simulink model "PH3_CSI_spv"  (R2017a)
settings: Solver=VariableStepAuto  StartTime=0.0  StopTime=10.0  MaxStep=1e-4  RelTol=1e-3
undefined symbols (not defined in the file): st_time3
libraries: powerlib x32, powerlib_meascontrol x6
settings Model: Creator=erich  LastModifiedBy=erich

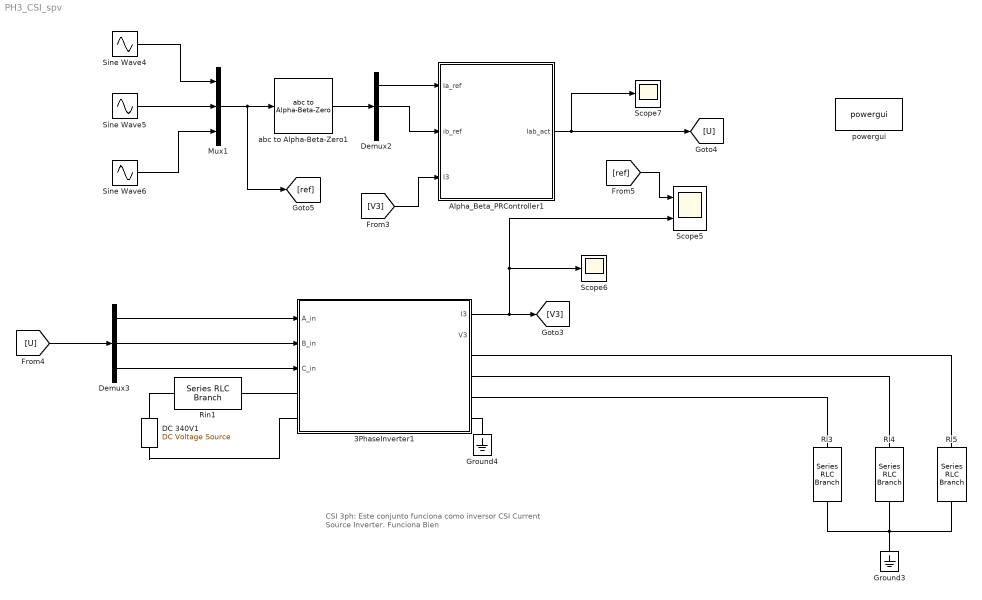
== system PH3_CSI_spv ==
  note: CSI 3ph:
      | Este conjunto funciona como inversor CSI
      | Current Source Inverter. Funciona Bien
  3PhaseInverter1 : Subsystem  mask{f_sw=10000, start_Delay=2e-3}
      mask prompts: f_sw "Switching Frequency (Hz)"; start_Delay "Time delay for drivers (s)"
      mask Display:
      | port_label('input', 1, 'A_u', 'texmode', 'on')
      | port_label('input', 2, 'B_u', 'texmode', 'on')
      | port_label('input', 3, 'C_u', 'texmode', 'on')
      | 
      | port_label('lconn', 1, 'DC +')
      | port_label('lconn', 2, 'DC -')
      | 
      | 
      | port_label('rconn', 1, 'A')
      | port_label('rconn', 2, 'B')
      | port_label('rconn', 3, 'C')
      | port_label('rconn', 4, 'Neutral')
      | 
      | port_label('output', 1, 'I_{3\Phi}', 'texmode', 'on')
      | port_label('output', 2, 'V_{3\Phi}', 'texmode', 'on')
      | 
      | plot([0.1 .9], [0.1 .9])
      | plot([0.2 .4], [.7 .7])
      | plot([0.2 .24], [.65 .65])
      | plot([0.28 .32], [.65 .65])
      | plot([0.36 .40], [.65 .65])
      | 
      | plot([.5:.01:.7], .25+sin(30*[.2:.01:.4])/10)
  Alpha_Beta_PRController1 : Subsystem  mask{Kp=50/100, Ki=25, w0=2*pi*60, wa=10}
      mask prompts: Kp "Ganancia Proporcional"; Ki "Ganancia Integral"; w0 "Frencuencia Central"; wa "Ancho de campana de resonancia"
      mask Display:
      | port_label('input', 1, '\fontsize{13} \alpha_{ref}', 'texmode', 'on')
      | port_label('input', 2, '\fontsize{13} \beta_{ref}', 'texmode', 'on')
      | port_label('input', 3, '\fontsize{13} [ a, b, c ]', 'texmode', 'on')
      | 
      | port_label('output', 1, '\fontsize{13} [ u_{a}, u_{b}, u_{c} ]', 'texmode', 'on')
      | 
      | 
      | %plot([.4 .6],.05+[.5 .7])
      | %plot([.4 .6],.05+[.9 .7])
      | %plot([.4 .4],.05+[.9 .5])
      | 
      | text(.53,.2,'\fontsize{25} \int', 'texmode', 'on')
      | plot(.65+[0:.01:pi/10], .2+sin(40*[0:.01:pi/10])/13)
      | 
      | %text(.5,.8,'\fontsize{15} PR_{\alpha \beta}', 'texmode', 'on')
  DC 340V1 : powerlib/Electrical Sources/DC Voltage Source  Amplitude=1000  Measurements=None
  Demux2 : Demux  Outputs=3
  Demux3 : Demux  Outputs=3
  Ground3 : powerlib/Elements/Ground  LConnTagsString=a
  Ground4 : powerlib/Elements/Ground  LConnTagsString=a
  Mux1 : Mux  Inputs=3
  Rin1 : powerlib/Elements/Series RLC Branch  LConnTagsString=__new0  RConnTagsString=__new0  BranchType=R  Resistance=.01  Inductance=0  SetiL0=off  InitialCurrent=0  Capacitance=0  Setx0=off  InitialVoltage=0  Measurements=None
  Rl3 : powerlib/Elements/Series RLC Branch  LConnTagsString=__new0  RConnTagsString=__new0  BranchType=R  Resistance=50  Inductance=1e-3  SetiL0=off  InitialCurrent=0  Capacitance=1e-6  Setx0=off  InitialVoltage=0  Measurements=None
  Rl4 : powerlib/Elements/Series RLC Branch  LConnTagsString=__new0  RConnTagsString=__new0  BranchType=R  Resistance=50  Inductance=1e-3  SetiL0=off  InitialCurrent=0  Capacitance=1e-6  Setx0=off  InitialVoltage=0  Measurements=None
  Rl5 : powerlib/Elements/Series RLC Branch  LConnTagsString=__new0  RConnTagsString=__new0  BranchType=R  Resistance=50  Inductance=1e-3  SetiL0=off  InitialCurrent=0  Capacitance=1e-6  Setx0=off  InitialVoltage=0  Measurements=None
  Scope5 : Scope  NumInputPorts=2
  Scope6 : Scope
  Scope7 : Scope
  Sine Wave4 : Sin  Amplitude=10  Frequency=2*pi*60
  Sine Wave5 : Sin  Amplitude=10  Frequency=2*pi*60  Phase=2*pi/3
  Sine Wave6 : Sin  Amplitude=10  Frequency=2*pi*60  Phase=-2*pi/3
  abc to Alpha-Beta-Zero1 : powerlib_meascontrol/Transformations/abc to Alpha-Beta-Zero
      settings: SourceProductName=Simscape Power Systems
  powergui : powerlib/powergui  Priority=1  SimulationMode=Continuous  SampleTime=50e-6  frequency=60  Iterations=50  frequencyindice=0  Pbase=100e6  ErrMax=1e-4  UnitsV=kV  UnitsW=MW  buscounter=0  FunctionMessages=off  echomessages=off  EnableUseOfTLC=off  CurrentSourceSwitches=off  DisableSnubberDevices=off  DisableRonSwitches=off  DisableVfSwitches=off  DisplayEquations=off  SolverType=Tustin/Backward Euler (TBE)  Interpol=off  ExternalGateDelay=off  methode=off  Ts=100  x0status=blocks  SPID=on  SwTol=0  HookPort=off  RestoreLinks=warning  ResistiveCurrentMeasurement=off  Frange=[0:2:500]  Ylog=off  Xlog=on  ShowGrid=off  save=off  variable=ZData  structure=0  ZoomFFT=off  StartTime=0.0  cycles=1  DisplayStyle=1  fundamental=60  FreqAxis=off  MaxFrequency=1000  frequencyindicesteady=1  RmsSteady=1  display=off
  wires:
  Demux3/3 -> 3PhaseInverter1/3(C_in)
  Demux2/2 -> Alpha_Beta_PRController1/2(ib_ref)
  Sine Wave4/1 -> Mux1/1
  3PhaseInverter1/1(I3) -> [V3], Scope6/1, Scope5/2
  Sine Wave6/1 -> Mux1/3
  [V3] -> Alpha_Beta_PRController1/3(I3)
  Mux1/1 -> abc to Alpha-Beta-Zero1/1, [ref]
  [ref] -> Scope5/1
  Demux2/1 -> Alpha_Beta_PRController1/1(Ia_ref)
  abc to Alpha-Beta-Zero1/1 -> Demux2/1
  Sine Wave5/1 -> Mux1/2
  Demux3/2 -> 3PhaseInverter1/2(B_in)
  Alpha_Beta_PRController1/1(Iab_act) -> [U], Scope7/1
  Demux3/1 -> 3PhaseInverter1/1(A_in)
  [U] -> Demux3/1
  connections:
  Rl4/RConn1 -- Rl5/RConn1 -- Ground3/LConn1 -- Rl3/RConn1
  Rl3/LConn1 -- 3PhaseInverter1/RConn3
  Rin1/RConn1 -- 3PhaseInverter1/LConn1
  Rl5/LConn1 -- 3PhaseInverter1/RConn1
  DC 340V1/RConn1 -- Rin1/LConn1
  Rl4/LConn1 -- 3PhaseInverter1/RConn2
  DC 340V1/LConn1 -- 3PhaseInverter1/LConn2
  3PhaseInverter1/RConn4 -- Ground4/LConn1

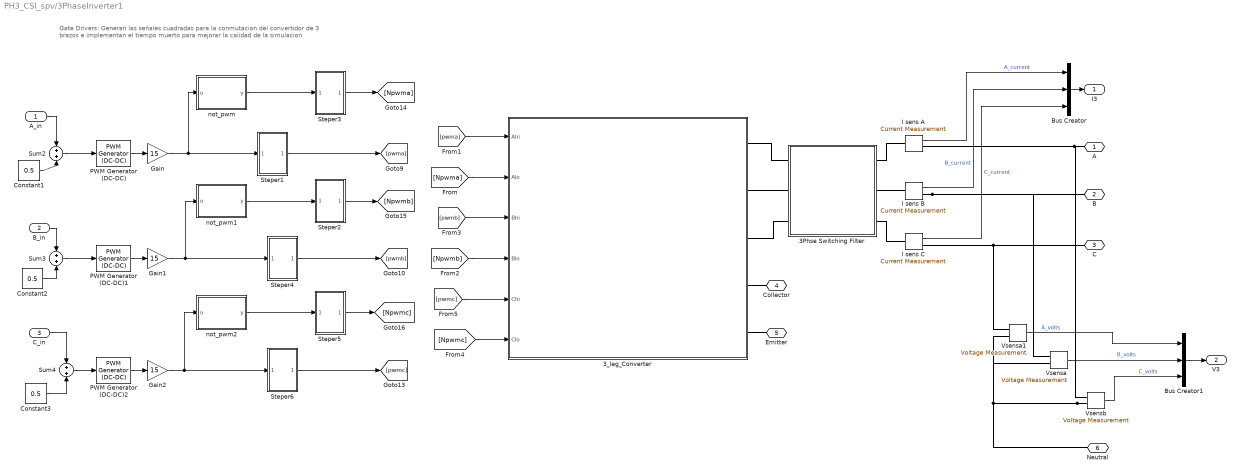
== system PH3_CSI_spv/3PhaseInverter1 ==
  note: Gate Drivers: Generan las señales cuadradas para
      | la conmutacion del convertidor de 3 brazos e implementan el
      | tiempo muerto para mejorar la calidad de la simulacion
  A_in : Inport
  B_in : Inport  Port=2
  C_in : Inport  Port=3
  3Phse Switching Filter : Subsystem
      mask Display:
      | port_label('lconn', 1, 'A_{in}', 'texmode', 'on')
      | port_label('lconn', 2, 'B_{in}', 'texmode', 'on')
      | port_label('lconn', 3, 'B_{in}', 'texmode', 'on')
      | port_label('rconn', 1, 'A_{out}', 'texmode', 'on')
      | port_label('rconn', 2, 'B_{out}', 'texmode', 'on')
      | port_label('rconn', 3, 'C_{out}', 'texmode', 'on')
      | 
      | 
      | plot([.2 .5], [.7 .7])
      | plot([.5 .6], [.7 .3])
      | plot([.6 .7], [.3 .3])
      | 
      | text(.2, .8, '\fontsize{12} H(\omega)', 'texmode', 'on')
      | text(.6, .25, '\fontsize{12} \omega', 'texmode', 'on')
  3_leg_Converter : Subsystem
      mask Display:
      | port_label('input', 1, 'Ahi')
      | port_label('input', 2, 'Alo')
      | port_label('input', 3, 'Bhi')
      | port_label('input', 4, 'Blo')
      | port_label('input', 5, 'Chi')
      | port_label('input', 6, 'Clo')
      | 
      | port_label('rconn', 1, 'A')
      | port_label('rconn', 2, 'B')
      | port_label('rconn', 3, 'C')
      | port_label('rconn', 4, 'Collector')
      | port_label('rconn', 5, 'Emitter')
      | 
      | lvx = [.1 .1];
      | lvy = [.1 .2];
      | lhx = [.1 .2];
      | lhy = [.1 .1];
      | 
      | 
      | % se dibujan los interruptores de la izquierda
      | plot(lvx+.07, lvy*.8+.028+.1)
      | plot(lvx+.1, lvy+.1)
      | plot(lhx*.5+.15, lhy+.1)
      | plot(lhx*.5+.15, lhy+.2)
      | plot(lhx*.5+.07, lhy+.15)
      | 
      | d=0.5;
      | 
      | plot(lvx+.07, lvy*.8+.028+.1+d)
      | plot(lvx+.1, lvy+.1+d)
      | plot(lhx*.5+.15, lhy+.1+d)
      | plot(lhx*.5+.15, lhy+.2+d)
      | plot(lhx*.5+.07, lhy+.15+d)
      | 
      | 
      | % se dibujan los interruptores del medio
      | h=.3;
      | 
      | plot(lvx+.07+h, lvy*.8+.028+.1)
      | plot(lvx+.1+h, lvy+.1)
      | plot(lhx*.5+.15+h, lhy+.1)
      | plot(lhx*.5+.15+h, lhy+.2)
      | plot(lhx*.5+.07+h, lhy+.15)
      | 
      | plot(lvx+.07+h, lvy*.8+.028+.1+d)
      | plot(lvx+.1+h, lvy+.1+d)
      | plot(lhx*.5+.15+h, lhy+.1+d)
      | plot(lhx*.5+.15+h, lhy+.2+d)
      | plot(lhx*.5+.07+h, lhy+.15+d)
      | 
      | % se dibujan los interruptores de la derecha
      | h=.6
      | 
      | plot(lvx+.07+h, lvy*.8+.028+.1)
      | plot(lvx+.1+h, lvy+.1)
      | plot(lhx*.5+.15+h, lhy+.1)
      | plot(lhx*.5+.15+h, lhy+.2)
      | plot(lhx*.5+.07+h, lhy+.15)
      | 
      | plot(lvx+.07+h, lvy*.8+.028+.1+d)
      | plot(lvx+.1+h, lvy+.1+d)
      | plot(lhx*.5+.15+h, lhy+.1+d)
      | plot(lhx*.5+.15+h, lhy+.2+d)
      | plot(lhx*.5+.07+h, lhy+.15+d)
      | 
      | 
      | % se conectan los interruptores.
      | plot(lvx+.15, lvy*4-.1)
      | plot(lvx+.15+.3, lvy*4-.1)
      | plot(lvx+.15+.6, lvy*4-.1)
      | 
      | 
      | plot(lvx+.15, lvy+.7)
      | plot(lvx+.15+.3, lvy+.7)
      | plot(lvx+.15+.6, lvy+.7)
      | 
      | plot(lvx+.15, lvy)
      | plot(lvx+.15+.3, lvy)
      | plot(lvx+.15+.6, lvy)
      | 
      | plot(lhx*6-.35, lhy)
      | plot(lhx*6-.35, lhy+.8)
      | 
      | % raul esteban alzate 313 515 86 11
  Bus Creator : BusCreator  Inputs='A_current','B_current','C_current'
  Bus Creator1 : BusCreator  Inputs='A_volts','B_volts','C_volts'
  Constant1 : Constant  Value=0.5
  Constant2 : Constant  Value=0.5
  Constant3 : Constant  Value=0.5
  Gain : Gain  Gain=15
  Gain1 : Gain  Gain=15
  Gain2 : Gain  Gain=15
  I sens A : powerlib/Measurements/Current Measurement  PhasorSimulation=off  OutputType=Complex  PSBequivalent=0
  I sens B : powerlib/Measurements/Current Measurement  PhasorSimulation=off  OutputType=Complex  PSBequivalent=0
  I sens C : powerlib/Measurements/Current Measurement  PhasorSimulation=off  OutputType=Complex  PSBequivalent=0
  PWM Generator (DC-DC) : powerlib_meascontrol/Pulse & Signal Generators/PWM Generator (DC-DC)  Fsw=f_sw  Ts=0
  PWM Generator (DC-DC)1 : powerlib_meascontrol/Pulse & Signal Generators/PWM Generator (DC-DC)  Fsw=f_sw  Ts=0
  PWM Generator (DC-DC)2 : powerlib_meascontrol/Pulse & Signal Generators/PWM Generator (DC-DC)  Fsw=f_sw  Ts=0
  Steper1 : Subsystem
  Steper2 : Subsystem
  Steper3 : Subsystem
  Steper4 : Subsystem
  Steper5 : Subsystem
  Steper6 : Subsystem
  Sum2 : Sum
  Sum3 : Sum
  Sum4 : Sum
  Vsensa : powerlib/Measurements/Voltage Measurement  PhasorSimulation=off  OutputType=Complex  PSBequivalent=0
  Vsensa1 : powerlib/Measurements/Voltage Measurement  PhasorSimulation=off  OutputType=Complex  PSBequivalent=0
  Vsensb : powerlib/Measurements/Voltage Measurement  PhasorSimulation=off  OutputType=Complex  PSBequivalent=0
  not_pwm : MATLAB Function  TreatAsAtomicUnit=on
  not_pwm1 : MATLAB Function  TreatAsAtomicUnit=on
  not_pwm2 : MATLAB Function  TreatAsAtomicUnit=on
  A : PMIOPort  Port=1  Side=Right
  B : PMIOPort  Port=2  Side=Right
  C : PMIOPort  Port=3  Side=Right
  Collector : PMIOPort  Port=4  Side=Left
  Emitter : PMIOPort  Port=5  Side=Left
  Neutral : PMIOPort  Port=6  Side=Right
  I3 : Outport
  V3 : Outport  Port=2
  wires:
  [Npwmc] -> 3_leg_Converter/6(Clo)
  [pwmc] -> 3_leg_Converter/5(Chi)
  [Npwmb] -> 3_leg_Converter/4(Blo)
  [pwmb] -> 3_leg_Converter/3(Bhi)
  [Npwma] -> 3_leg_Converter/2(Alo)
  [pwma] -> 3_leg_Converter/1(Ahi)
  Vsensa1/1 -> Bus Creator1/1  "A_volts"
  Vsensa/1 -> Bus Creator1/2  "B_volts"
  Bus Creator1/1 -> V3/1
  Vsensb/1 -> Bus Creator1/3  "C_volts"
  Steper6/1(Out1) -> [pwmc]
  Gain/1 -> not_pwm/1(u), Steper1/1(In1)
  Steper3/1(Out1) -> [Npwma]
  Constant2/1 -> Sum3/2
  I sens B/1 -> Bus Creator/2  "B_current"
  Steper1/1(Out1) -> [pwma]
  Steper5/1(Out1) -> [Npwmc]
  Gain2/1 -> not_pwm2/1(u), Steper6/1(In1)
  Sum3/1 -> PWM Generator (DC-DC)1/1
  Bus Creator/1 -> I3/1
  I sens A/1 -> Bus Creator/1  "A_current"
  A_in/1 -> Sum2/1
  Steper2/1(Out1) -> [Npwmb]
  Constant1/1 -> Sum2/2
  B_in/1 -> Sum3/1
  PWM Generator (DC-DC)/1 -> Gain/1
  I sens C/1 -> Bus Creator/3  "C_current"
  Sum2/1 -> PWM Generator (DC-DC)/1
  C_in/1 -> Sum4/1
  not_pwm2/1(y) -> Steper5/1(In1)
  PWM Generator (DC-DC)1/1 -> Gain1/1
  Constant3/1 -> Sum4/2
  not_pwm/1(y) -> Steper3/1(In1)
  Sum4/1 -> PWM Generator (DC-DC)2/1
  PWM Generator (DC-DC)2/1 -> Gain2/1
  not_pwm1/1(y) -> Steper2/1(In1)
  Gain1/1 -> not_pwm1/1(u), Steper4/1(In1)
  Steper4/1(Out1) -> [pwmb]
  connections:
  3_leg_Converter/RConn5 -- Emitter/RConn1
  3_leg_Converter/RConn4 -- Collector/RConn1
  Vsensb/LConn2 -- Vsensa1/LConn2 -- Vsensa/LConn2 -- Neutral/RConn1
  I sens C/LConn1 -- 3Phse Switching Filter/RConn3
  C/RConn1 -- I sens C/RConn1 -- Vsensa1/LConn1
  3Phse Switching Filter/LConn1 -- 3_leg_Converter/RConn1
  I sens B/RConn1 -- Vsensa/LConn1 -- B/RConn1
  I sens A/LConn1 -- 3Phse Switching Filter/RConn1
  3Phse Switching Filter/LConn3 -- 3_leg_Converter/RConn3
  A/RConn1 -- I sens A/RConn1 -- Vsensb/LConn1
  I sens B/LConn1 -- 3Phse Switching Filter/RConn2
  3Phse Switching Filter/LConn2 -- 3_leg_Converter/RConn2

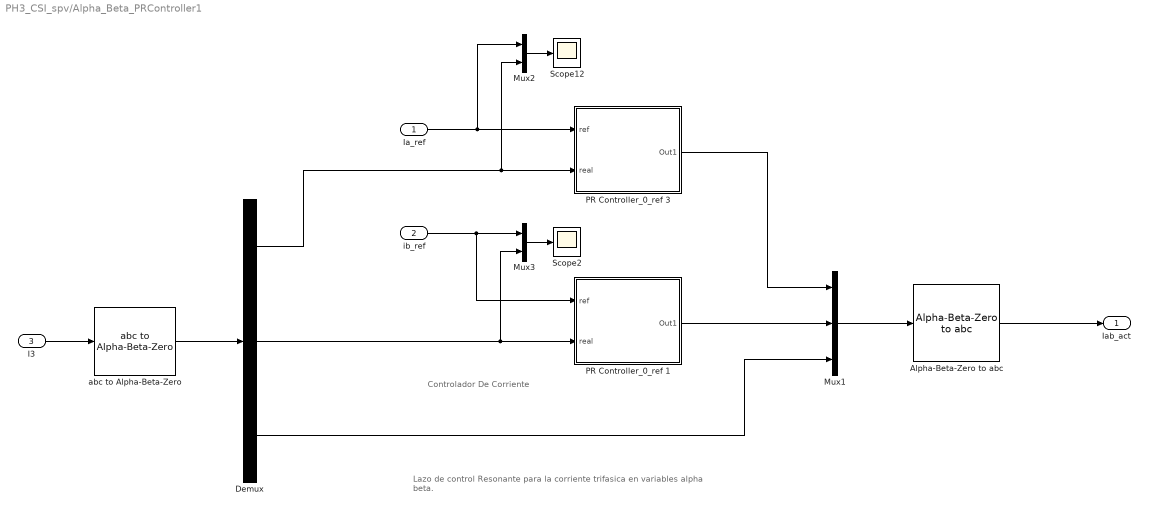
== system PH3_CSI_spv/Alpha_Beta_PRController1 ==
  note: Lazo de control Resonante para la
      | corriente trifasica en variables alpha beta.
  note: Controlador De Corriente
  Ia_ref : Inport
  ib_ref : Inport  Port=2
  I3 : Inport  Port=3
  Alpha-Beta-Zero to abc : powerlib_meascontrol/Transformations/Alpha-Beta-Zero to abc
      settings: SourceProductName=Simscape Power Systems  SourceProductBaseCode=PS
  Demux : Demux  Outputs=3
  Mux1 : Mux  Inputs=3
  Mux2 : Mux  Inputs=2
  Mux3 : Mux  Inputs=2
  PR Controller_0_ref 1 : Subsystem  mask{Kp=Kp, Ki=Ki, wa=wa, w0=w0}
      mask prompts: Kp "Ganancia Proporcional"; Ki "Ganancia Integral"; wa "Ancho camapana resonancia"; w0 "Frecuencia Central"
      mask Display:
      | port_label('input',1,'ref')
      | port_label('input',2,'sens')
      | port_label('output',1,'out')
      | 
      | plot(.4+[0:.01:pi/10], .32+sin(40*[0:.01:pi/10])/13)
      | 
      | plot([.4 .6],.05+[.5 .7])
      | plot([.4 .6],.05+[.9 .7])
      | plot([.4 .4],.05+[.9 .5])
      | 
      | text(.27,.37,'\fontsize{25} \int', 'texmode', 'on')
  PR Controller_0_ref 3 : Subsystem  mask{Kp=Kp, Ki=Ki, wa=wa, w0=w0}
      mask prompts: Kp "Ganancia Proporcional"; Ki "Ganancia Integral"; wa "Ancho camapana resonancia"; w0 "Frecuencia Central"
      mask Display:
      | port_label('input',1,'ref')
      | port_label('input',2,'sens')
      | port_label('output',1,'out')
      | 
      | plot(.4+[0:.01:pi/10], .32+sin(40*[0:.01:pi/10])/13)
      | 
      | plot([.4 .6],.05+[.5 .7])
      | plot([.4 .6],.05+[.9 .7])
      | plot([.4 .4],.05+[.9 .5])
      | 
      | text(.27,.37,'\fontsize{25} \int', 'texmode', 'on')
  Scope12 : Scope
  Scope2 : Scope
  abc to Alpha-Beta-Zero : powerlib_meascontrol/Transformations/abc to Alpha-Beta-Zero
      settings: SourceProductName=Simscape Power Systems
  Iab_act : Outport
  wires:
  Demux/1 -> PR Controller_0_ref 3/2(real), Mux2/2
  Demux/3 -> Mux1/3
  PR Controller_0_ref 3/1(Out1) -> Mux1/1
  Ia_ref/1 -> PR Controller_0_ref 3/1(ref), Mux2/1
  ib_ref/1 -> Mux3/1, PR Controller_0_ref 1/1(ref)
  abc to Alpha-Beta-Zero/1 -> Demux/1
  Alpha-Beta-Zero to abc/1 -> Iab_act/1
  Mux3/1 -> Scope2/1
  Mux1/1 -> Alpha-Beta-Zero to abc/1
  PR Controller_0_ref 1/1(Out1) -> Mux1/2
  Demux/2 -> Mux3/2, PR Controller_0_ref 1/2(real)
  Mux2/1 -> Scope12/1
  I3/1 -> abc to Alpha-Beta-Zero/1

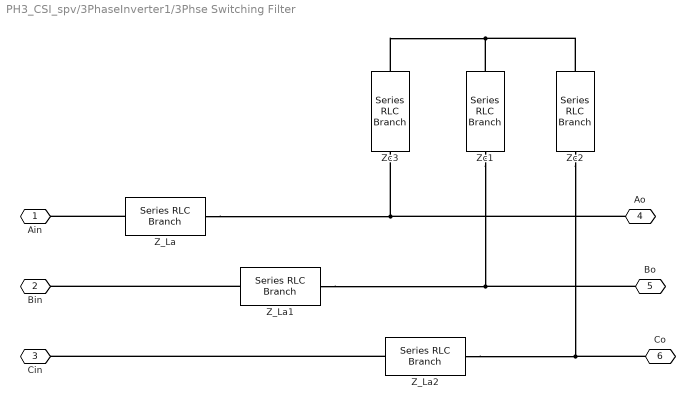
== system PH3_CSI_spv/3PhaseInverter1/3Phse Switching Filter ==
  Z_La : powerlib/Elements/Series RLC Branch  LConnTagsString=__new0  RConnTagsString=__new0  BranchType=RL  Resistance=.01  Inductance=4e-3  SetiL0=off  InitialCurrent=0  Capacitance=2.2e-6  Setx0=off  InitialVoltage=0  Measurements=None
  Z_La1 : powerlib/Elements/Series RLC Branch  LConnTagsString=__new0  RConnTagsString=__new0  BranchType=RL  Resistance=.1  Inductance=4e-3  SetiL0=off  InitialCurrent=0  Capacitance=2.2e-6  Setx0=off  InitialVoltage=0  Measurements=None
  Z_La2 : powerlib/Elements/Series RLC Branch  LConnTagsString=__new0  RConnTagsString=__new0  BranchType=RL  Resistance=.1  Inductance=4e-3  SetiL0=off  InitialCurrent=0  Capacitance=2.2e-6  Setx0=off  InitialVoltage=0  Measurements=None
  Zc1 : powerlib/Elements/Series RLC Branch  LConnTagsString=__new0  RConnTagsString=__new0  BranchType=RC  Resistance=1e-3  Inductance=1e-9  SetiL0=off  InitialCurrent=0  Capacitance=2.2e-6  Setx0=off  InitialVoltage=0  Measurements=None
  Zc2 : powerlib/Elements/Series RLC Branch  LConnTagsString=__new0  RConnTagsString=__new0  BranchType=RC  Resistance=1e-3  Inductance=1e-9  SetiL0=off  InitialCurrent=0  Capacitance=2.2e-6  Setx0=off  InitialVoltage=0  Measurements=None
  Zc3 : powerlib/Elements/Series RLC Branch  LConnTagsString=__new0  RConnTagsString=__new0  BranchType=RC  Resistance=1e-3  Inductance=1e-9  SetiL0=off  InitialCurrent=0  Capacitance=2.2e-6  Setx0=off  InitialVoltage=0  Measurements=None
  Ain : PMIOPort  Port=1  Side=Left
  Bin : PMIOPort  Port=2  Side=Left
  Cin : PMIOPort  Port=3  Side=Left
  Ao : PMIOPort  Port=4  Side=Right
  Bo : PMIOPort  Port=5  Side=Right
  Co : PMIOPort  Port=6  Side=Right
  connections:
  Z_La2/LConn1 -- Cin/RConn1
  Z_La1/LConn1 -- Bin/RConn1
  Z_La/LConn1 -- Ain/RConn1
  Z_La/RConn1 -- Zc3/LConn1 -- Ao/RConn1
  Z_La2/RConn1 -- Co/RConn1 -- Zc2/LConn1
  Z_La1/RConn1 -- Zc1/LConn1 -- Bo/RConn1
  Zc2/RConn1 -- Zc1/RConn1 -- Zc3/RConn1

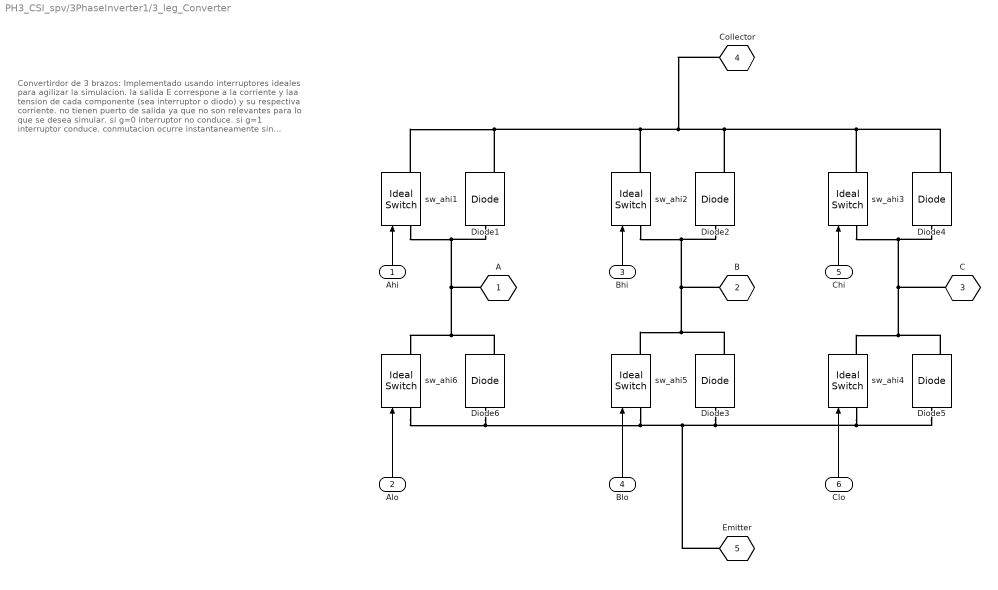
== system PH3_CSI_spv/3PhaseInverter1/3_leg_Converter ==
  note: Convertirdor de 3 brazos:
      |
      | Implementado usando interruptores
      | ideales para agilizar la simulacion.
      | la salida E correspone a la corriente y laa
      | tension de cada componente
      | (sea interruptor o diodo) y su respectiva
      | corriente. no tienen puerto de salida ya que no
      | son relevantes para lo que se desea simular.
      |
      | si g=0 interruptor no conduce.
      | si g=1 interruptor conduce.
      |
      | conmutacion ocurre instantaneamente sin
      | retardo.
  Ahi : Inport
  Alo : Inport  Port=2
  Bhi : Inport  Port=3
  Blo : Inport  Port=4
  Chi : Inport  Port=5
  Clo : Inport  Port=6
   sw_ahi{1..6} (6 alike) : powerlib/Power Electronics/Ideal Switch  Ron=20e-3  Lon=0  IC=0  Rs=1e6  Cs=10e-12  Measurements=on
  Diode{1..6} (6 alike) : powerlib/Power Electronics/Diode  Ron=.2  Lon=0  Vf=0.8  IC=0  UseSnubber=0  Rs=0  Cs=0  Measurements=on
  " A" : PMIOPort  Tag=PMCPort  Port=1  Side=Right
  B : PMIOPort  Tag=PMCPort  Port=2  Side=Right
  C : PMIOPort  Tag=PMCPort  Port=3  Side=Right
  Collector : PMIOPort  Tag=PMCPort  Port=4  Side=Right
  Emitter : PMIOPort  Tag=PMCPort  Port=5  Side=Right
  wires:
  Chi/1 -> " sw_ahi3"/1
  Bhi/1 -> " sw_ahi2"/1
  Blo/1 -> " sw_ahi5"/1
  Ahi/1 -> " sw_ahi1"/1
  Alo/1 -> " sw_ahi6"/1
  Clo/1 -> " sw_ahi4"/1
  connections:
  " sw_ahi4"/RConn1 -- Diode5/RConn1 -- Diode4/LConn1 -- " sw_ahi3"/LConn1 -- C/RConn1
  " sw_ahi1"/LConn1 -- Diode1/LConn1 -- " A"/RConn1 -- Diode6/RConn1 -- " sw_ahi6"/RConn1
  " sw_ahi3"/RConn1 -- Diode4/RConn1 -- Diode1/RConn1 -- " sw_ahi1"/RConn1 -- " sw_ahi2"/RConn1 -- Collector/RConn1 -- Diode2/RConn1
  " sw_ahi5"/LConn1 -- " sw_ahi6"/LConn1 -- Diode6/LConn1 -- Emitter/RConn1 -- Diode5/LConn1 -- " sw_ahi4"/LConn1 -- Diode3/LConn1
  " sw_ahi5"/RConn1 -- Diode2/LConn1 -- " sw_ahi2"/LConn1 -- B/RConn1 -- Diode3/RConn1

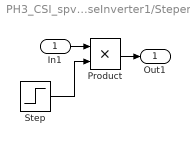
== system PH3_CSI_spv/3PhaseInverter1/Steper1 ==
  In1 : Inport
  Product : Product
  Step : Step  Time=start_Delay  SampleTime=0
  Out1 : Outport
  wires:
  Product/1 -> Out1/1
  In1/1 -> Product/1
  Step/1 -> Product/2

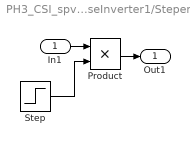
== system PH3_CSI_spv/3PhaseInverter1/Steper2 ==
  In1 : Inport
  Product : Product
  Step : Step  Time=start_Delay  SampleTime=0
  Out1 : Outport
  wires:
  Step/1 -> Product/2
  In1/1 -> Product/1
  Product/1 -> Out1/1

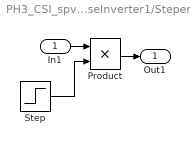
== system PH3_CSI_spv/3PhaseInverter1/Steper3 ==
  In1 : Inport
  Product : Product
  Step : Step  Time=start_Delay  SampleTime=0
  Out1 : Outport
  wires:
  Step/1 -> Product/2
  In1/1 -> Product/1
  Product/1 -> Out1/1

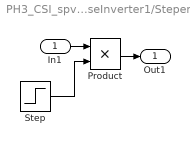
== system PH3_CSI_spv/3PhaseInverter1/Steper4 ==
  In1 : Inport
  Product : Product
  Step : Step  Time=start_Delay  SampleTime=0
  Out1 : Outport
  wires:
  Product/1 -> Out1/1
  In1/1 -> Product/1
  Step/1 -> Product/2

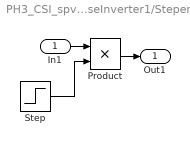
== system PH3_CSI_spv/3PhaseInverter1/Steper5 ==
  In1 : Inport
  Product : Product
  Step : Step  Time=start_Delay  SampleTime=0
  Out1 : Outport
  wires:
  Step/1 -> Product/2
  In1/1 -> Product/1
  Product/1 -> Out1/1

== system PH3_CSI_spv/3PhaseInverter1/Steper6 ==
  In1 : Inport
  Product : Product
  Step : Step  Time=start_Delay  SampleTime=0
  Out1 : Outport
  wires:
  Product/1 -> Out1/1
  In1/1 -> Product/1
  Step/1 -> Product/2

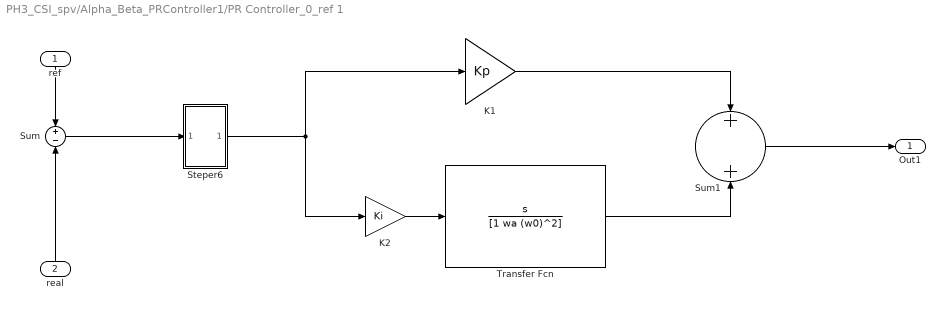
== system PH3_CSI_spv/Alpha_Beta_PRController1/PR Controller_0_ref 1 ==
  ref : Inport
  real : Inport  Port=2
  K1 : Gain  Gain=Kp
  K2 : Gain  Gain=Ki
  Steper6 : Subsystem
  Sum : Sum  Inputs=+-
  Sum1 : Sum  Inputs=+|+
  Transfer Fcn : TransferFcn  Numerator=[1 0]  Denominator=[1 wa (w0)^2]
  Out1 : Outport
  wires:
  real/1 -> Sum/2
  ref/1 -> Sum/1
  Sum/1 -> Steper6/1(In1)
  K1/1 -> Sum1/1
  Transfer Fcn/1 -> Sum1/2
  K2/1 -> Transfer Fcn/1
  Steper6/1(Out1) -> K1/1, K2/1
  Sum1/1 -> Out1/1

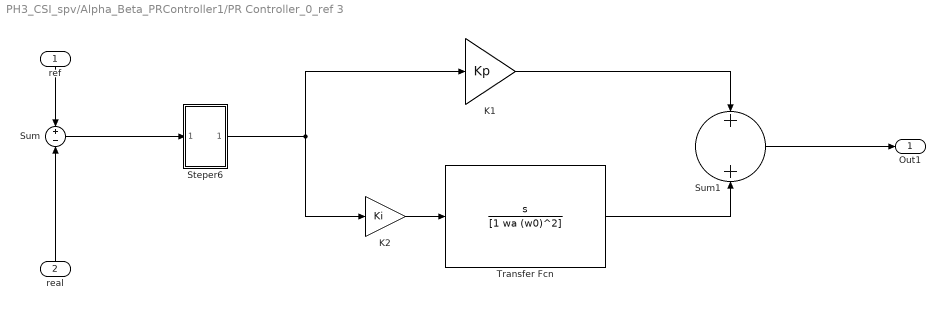
== system PH3_CSI_spv/Alpha_Beta_PRController1/PR Controller_0_ref 3 ==
  ref : Inport
  real : Inport  Port=2
  K1 : Gain  Gain=Kp
  K2 : Gain  Gain=Ki
  Steper6 : Subsystem
  Sum : Sum  Inputs=+-
  Sum1 : Sum  Inputs=+|+
  Transfer Fcn : TransferFcn  Numerator=[1 0]  Denominator=[1 wa (w0)^2]
  Out1 : Outport
  wires:
  Sum1/1 -> Out1/1
  Steper6/1(Out1) -> K2/1, K1/1
  K2/1 -> Transfer Fcn/1
  Transfer Fcn/1 -> Sum1/2
  K1/1 -> Sum1/1
  Sum/1 -> Steper6/1(In1)
  ref/1 -> Sum/1
  real/1 -> Sum/2

== system PH3_CSI_spv/Alpha_Beta_PRController1/PR Controller_0_ref 1/Steper6 ==
  In1 : Inport
  Product : Product
  Step : Step  Time=st_time3  SampleTime=0
  Out1 : Outport
  wires:
  Product/1 -> Out1/1
  In1/1 -> Product/1
  Step/1 -> Product/2

== system PH3_CSI_spv/Alpha_Beta_PRController1/PR Controller_0_ref 3/Steper6 ==
  In1 : Inport
  Product : Product
  Step : Step  Time=st_time3  SampleTime=0
  Out1 : Outport
  wires:
  Step/1 -> Product/2
  In1/1 -> Product/1
  Product/1 -> Out1/1

== matlab function PH3_CSI_spv/3PhaseInverter1/not_pwm ==
  data: u input; y output
function y = fcn(u)
%#codegen

if(u==0 || u<0)
    a=15;
else
    a=0;
end;

y = a;

== matlab function PH3_CSI_spv/3PhaseInverter1/not_pwm1 ==
  data: u input; y output
function y = fcn(u)
%#codegen

if(u==0 || u<0)
    a=5;
else
    a=0;
end;

y = a;

== matlab function PH3_CSI_spv/3PhaseInverter1/not_pwm2 ==
  data: u input; y output
function y = fcn(u)
%#codegen

if(u==0 || u<0)
    a=5;
else
    a=0;
end;

y = a;
